simulink subsystem "MSD_Estimator_ASY"  (R2022a)
settings: Solver=VariableStepAuto  StartTime=0.0  StopTime=10.0  RelTol=1e-3
values from neighbouring files (symbols this model uses):
  A_DT = SS_DT.A    [KalmanTesting_Mechanical.m]    (also in KalmanTesting_Mechanical_DataGeneration.m; KalmanTesting_Mechanical_InputQ_Sine.m; KalmanTesting_Mechanical_InputQ_Step.m; KalmanTesting_Mechanical_InputQ_Step_DataGen.m)
  B_DT = SS_DT.B    [KalmanTesting_Mechanical.m]    (also in KalmanTesting_Mechanical_DataGeneration.m; KalmanTesting_Mechanical_InputQ_Sine.m; KalmanTesting_Mechanical_InputQ_Step.m; KalmanTesting_Mechanical_InputQ_Step_DataGen.m)
  C = [1 0 0 0]    [KalmanTesting_Mechanical.m]    (also in KalmanTesting_Mechanical_DataGeneration.m = [0 0 0 1]; KalmanTesting_Mechanical_InputQ_Sine.m = [0 0 0 1]; KalmanTesting_Mechanical_InputQ_Step.m; KalmanTesting_Mechanical_InputQ_Step_DataGen.m = [0 0 0 1])
  K_infty = P_infty*C'*inv(C*P_infty*C' + R)    [KalmanTesting_Mechanical.m]    (also in KalmanTesting_Mechanical_DataGeneration.m; KalmanTesting_Mechanical_InputQ_Sine.m; KalmanTesting_Mechanical_InputQ_Step.m; KalmanTesting_Mechanical_InputQ_Step_DataGen.m)
  Ts = .1    (= 0.1)    [KalmanTesting_Mechanical.m]    (also in KalmanTesting_Mechanical_DataGeneration.m = TT; KalmanTesting_Mechanical_InputQ_Sine.m = 1/SIM.fq/25; KalmanTesting_Mechanical_InputQ_Step.m; KalmanTesting_Mechanical_InputQ_Step_DataGen.m = TT)
  x_0_est = [0;0;0;0]    [KalmanTesting_Mechanical_InputQ_Sine.m]    (also in KalmanTesting_Mechanical_InputQ_Step.m; KalmanTesting_Mechanical_InputQ_Step_DataGen.m)
settings Model: Creator=tyevans  LastModifiedBy=tyevans

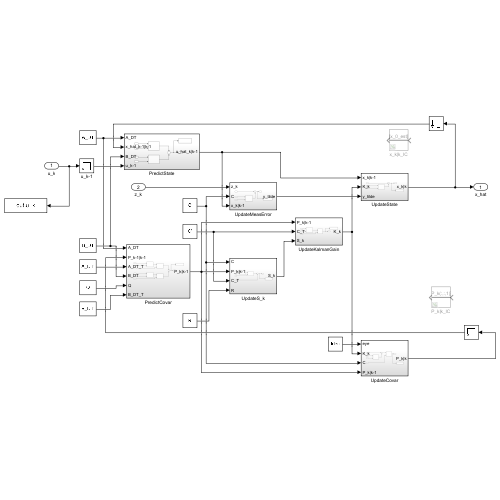
[thumbnail: Simulink's stored preview of the top-level diagram]
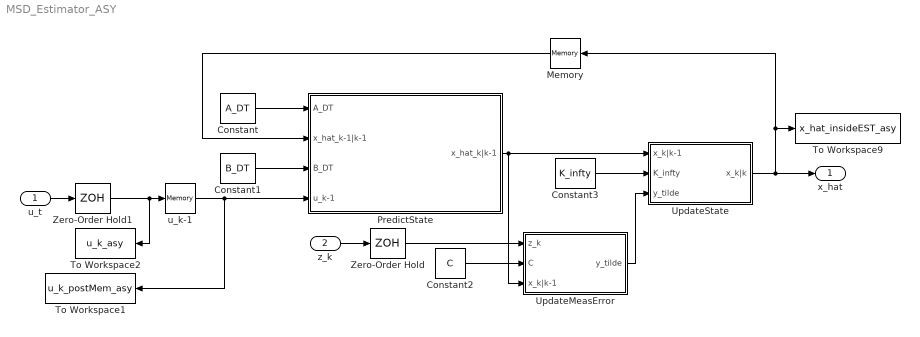
== system MSD_Estimator_ASY ==
  u_t : Inport
  z_k : Inport  Port=2
  Constant : Constant  Value=A_DT  VectorParams1D=off
  Constant1 : Constant  Value=B_DT  VectorParams1D=off
  Constant2 : Constant  Value=C  VectorParams1D=off
  Constant3 : Constant  Value=K_infty  VectorParams1D=off
  Memory : Memory  InitialCondition=x_0_est  InheritSampleTime=on
  PredictState : Subsystem
  To Workspace1 : ToWorkspace  VariableName=u_k_postMem_asy  SaveFormat=Structure With Time  SampleTime=-1
  To Workspace2 : ToWorkspace  VariableName=u_k_asy  SaveFormat=Structure With Time  SampleTime=-1
  To Workspace9 : ToWorkspace  VariableName=x_hat_insideEST_asy  SaveFormat=Structure With Time  SampleTime=-1
  UpdateMeasError : Subsystem
  UpdateState : Subsystem
  Zero-Order Hold : ZeroOrderHold  SampleTime=Ts
  Zero-Order Hold1 : ZeroOrderHold  SampleTime=Ts
  u_k-1 : Memory  InheritSampleTime=on
  x_hat : Outport
  wires:
  Constant3/1 -> UpdateState/2(K_infty)
  Constant1/1 -> PredictState/3(B_DT)
  Zero-Order Hold/1 -> UpdateMeasError/1(z_k)
  u_t/1 -> Zero-Order Hold1/1
  u_k-1/1 -> To Workspace1/1, PredictState/4(u_k-1)
  z_k/1 -> Zero-Order Hold/1
  UpdateMeasError/1(y_tilde) -> UpdateState/3(y_tilde)
  Constant/1 -> PredictState/1(A_DT)
  Constant2/1 -> UpdateMeasError/2(C)
  Memory/1 -> PredictState/2(x_hat_k-1|k-1)
  Zero-Order Hold1/1 -> u_k-1/1, To Workspace2/1
  UpdateState/1(x_k|k) -> x_hat/1, Memory/1, To Workspace9/1
  PredictState/1(x_hat_k|k-1) -> UpdateState/1(x_k|k-1), UpdateMeasError/3(x_k|k-1)

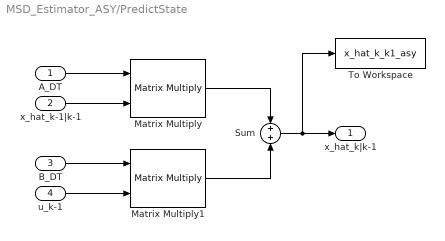
== system MSD_Estimator_ASY/PredictState ==
  A_DT : Inport
  x_hat_k-1|k-1 : Inport  Port=2
  B_DT : Inport  Port=3
  u_k-1 : Inport  Port=4
  Matrix Multiply : Product  Multiplication=Matrix(*)
  Matrix Multiply1 : Product  Multiplication=Matrix(*)
  Sum : Sum
  To Workspace : ToWorkspace  VariableName=x_hat_k_k1_asy  SaveFormat=Structure With Time  SampleTime=-1
  x_hat_k|k-1 : Outport
  wires:
  Sum/1 -> x_hat_k|k-1/1, To Workspace/1
  Matrix Multiply1/1 -> Sum/2
  Matrix Multiply/1 -> Sum/1
  u_k-1/1 -> Matrix Multiply1/2
  B_DT/1 -> Matrix Multiply1/1
  x_hat_k-1|k-1/1 -> Matrix Multiply/2
  A_DT/1 -> Matrix Multiply/1

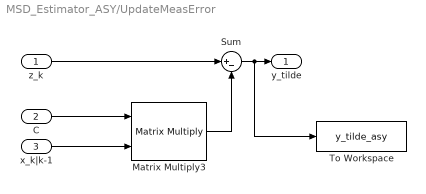
== system MSD_Estimator_ASY/UpdateMeasError ==
  z_k : Inport
  C : Inport  Port=2
  x_k|k-1 : Inport  Port=3
  Matrix Multiply3 : Product  Multiplication=Matrix(*)
  Sum : Sum  Inputs=|+-
  To Workspace : ToWorkspace  VariableName=y_tilde_asy  SaveFormat=Structure With Time  SampleTime=-1
  y_tilde : Outport
  wires:
  C/1 -> Matrix Multiply3/1
  x_k|k-1/1 -> Matrix Multiply3/2
  z_k/1 -> Sum/1
  Sum/1 -> y_tilde/1, To Workspace/1
  Matrix Multiply3/1 -> Sum/2

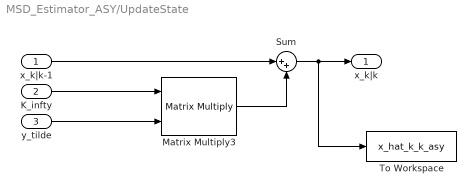
== system MSD_Estimator_ASY/UpdateState ==
  x_k|k-1 : Inport
  K_infty : Inport  Port=2
  y_tilde : Inport  Port=3
  Matrix Multiply3 : Product  Multiplication=Matrix(*)
  Sum : Sum  Inputs=|++
  To Workspace : ToWorkspace  VariableName=x_hat_k_k_asy  SaveFormat=Structure With Time  SampleTime=-1
  x_k|k : Outport
  wires:
  Sum/1 -> x_k|k/1, To Workspace/1
  Matrix Multiply3/1 -> Sum/2
  x_k|k-1/1 -> Sum/1
  y_tilde/1 -> Matrix Multiply3/2
  K_infty/1 -> Matrix Multiply3/1
